simulink model "mass_springg"  (R2021a)
settings: Solver=VariableStepAuto  StartTime=0.0  StopTime=25  MaxStep=0.005  RelTol=1e-3
values from neighbouring files (symbols this model uses):
  A = adj    [ceren_function.m]    (also in deneme.m = [A_1 ;A_2; A_3;A_4; A_5;A_6])
  B = [B_1; B_2; B_3; B_4; B_5; B_6]    [deneme.m]
  B_dist = 2*[0; 0.0717; 0; -0.7374; 0; 1.9776]    [deneme.m]
  C1 = [0.0717 0 -0.7374 0 1.9776 0]    [deneme.m]
  C2 = [0.0699 0 -0.5958 0 1.2029 0]    [deneme.m]
  C3 = [0.0665 0 -0.4444 0 0.4020 0]    [deneme.m]
  C4 = [0.0630 0 -0.2977 0 -0.3216 0]    [deneme.m]
  D = [0 0 0 0]    [deneme.m]
  K = kron(A, B)    [kronecker.m]
  w1 = 2*pi* 0.2745    (= 1.72473436682)    [deneme.m]
  w2 = 2*pi* 2.9446    (= 18.5014674555)    [deneme.m]
settings Model: PacingRate=9  Creator=umut  LastModifiedBy=umut

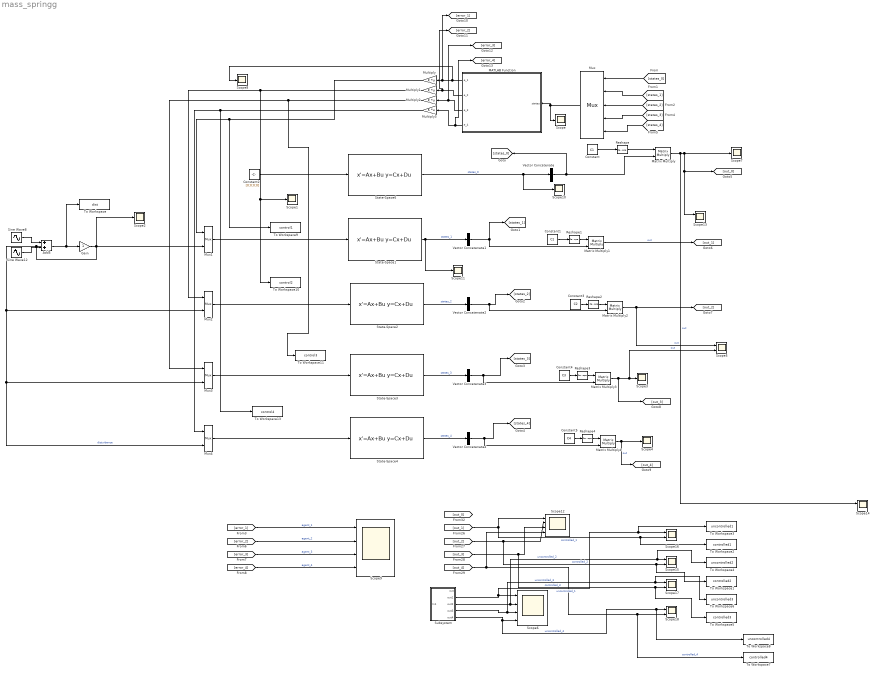
== system mass_springg ==
  Add5 : Sum
  Constant : Constant  Value=C1
  Constant1 : Constant  Value=C1
  Constant2 : Constant  Value=[0;0;0;0]
  Constant3 : Constant  Value=C2
  Constant4 : Constant  Value=C3
  Constant5 : Constant  Value=C4
  Gain : Gain
  MATLAB Function : MATLAB Function  TreatAsAtomicUnit=on
  Matrix Multiply{,1..4} (5 alike) : Product  Multiplication=Matrix(*)
  Multiply{,1..3} (4 alike) : Gain  Gain=K  Multiplication=Matrix(K*u)
  Mux : Mux  Inputs=5
  Mux{1..4} (4 alike) : Mux  Inputs=2
  Reshape{,1..4} (5 alike) : Reshape  OutputDimensionality=Customize  OutputDimensions=[1,6]
  Scope{,1..4,7..8,10..11} (9 alike) : Scope
  Scope12 : Scope  NumInputPorts=4
  Scope{5,13..18} (7 alike) : Scope  NumInputPorts=2
  Scope6 : Scope  NumInputPorts=4
  Scope9 : Scope  NumInputPorts=4
  Sine Wave12 : Sin  Amplitude=0.5  Frequency=w2  SampleTime=0
  Sine Wave8 : Sin  Amplitude=0.5  Frequency=w1  SampleTime=0
  State-Space1 : StateSpace  A=A  B=[B B_dist]  C=eye(6)  D=[D 0;D 0;D 0;D 0;D 0;D 0]  InitialCondition=[0.1;0.2;0.3;0.4;0.5;0.6]
  State-Space2 : StateSpace  A=A  B=[B B_dist]  C=eye(6)  D=[D 0;D 0;D 0;D 0;D 0;D 0]  InitialCondition=[0.6;0.5;0.4;0.3;0.2;0.1]
  State-Space3 : StateSpace  A=A  B=[B B_dist]  C=eye(6)  D=[D 0;D 0;D 0;D 0;D 0;D 0]  InitialCondition=[0.6;0.3;0.1;0.4;0;0.8]
  State-Space4 : StateSpace  A=A  B=[B B_dist]  C=eye(6)  D=[D 0;D 0;D 0;D 0;D 0;D 0]  InitialCondition=[0.3;0.1;0.7;0.2;0.8;0.4]
  State-Space6 : StateSpace  A=A  B=B  C=zeros(6)  D=[D;D;D;D;D;D]  InitialCondition=[0.1;0.2;0.3;0.4;0.5;0.6]
  Subsystem : Subsystem
  To Workspace : ToWorkspace  VariableName=dist  SampleTime=-1
      settings: Save2DSignal=2-D array (concatenate along first dimension)
  To Workspace1 : ToWorkspace  VariableName=controlled2  SampleTime=-1
      settings: Save2DSignal=2-D array (concatenate along first dimension)
  To Workspace10 : ToWorkspace  VariableName=control2  SampleTime=-1
      settings: Save2DSignal=2-D array (concatenate along first dimension)
  To Workspace11 : ToWorkspace  VariableName=control3  SampleTime=-1
      settings: Save2DSignal=2-D array (concatenate along first dimension)
  To Workspace13 : ToWorkspace  VariableName=control4  SampleTime=-1
      settings: Save2DSignal=2-D array (concatenate along first dimension)
  To Workspace2 : ToWorkspace  VariableName=controlled1  SampleTime=-1
      settings: Save2DSignal=2-D array (concatenate along first dimension)
  To Workspace3 : ToWorkspace  VariableName=uncontrolled1  SampleTime=-1
      settings: Save2DSignal=2-D array (concatenate along first dimension)
  To Workspace4 : ToWorkspace  VariableName=uncontrolled2  SampleTime=-1
      settings: Save2DSignal=2-D array (concatenate along first dimension)
  To Workspace5 : ToWorkspace  VariableName=controlled3  SampleTime=-1
      settings: Save2DSignal=2-D array (concatenate along first dimension)
  To Workspace6 : ToWorkspace  VariableName=uncontrolled3  SampleTime=-1
      settings: Save2DSignal=2-D array (concatenate along first dimension)
  To Workspace7 : ToWorkspace  VariableName=controlled4  SampleTime=-1
      settings: Save2DSignal=2-D array (concatenate along first dimension)
  To Workspace8 : ToWorkspace  VariableName=uncontrolled4  SampleTime=-1
      settings: Save2DSignal=2-D array (concatenate along first dimension)
  To Workspace9 : ToWorkspace  VariableName=control1  SampleTime=-1
      settings: Save2DSignal=2-D array (concatenate along first dimension)
  Vector Concatenate{,1..4} (5 alike) : Concatenate  NumInputs=1  Mode=Multidimensional array  ConcatenateDimension=4
  wires:
  State-Space1/1 -> Vector Concatenate1/1, Scope11/1  "states_1"
  Mux/1 -> Scope/1, MATLAB Function/1(states)
  State-Space2/1 -> Vector Concatenate2/1  "states_2"
  Matrix Multiply2/1 -> [out_2], Scope5/1  "out"
  Matrix Multiply3/1 -> [out_3], Scope5/2, Scope3/1  "out"
  State-Space3/1 -> Vector Concatenate3/1  "states_3"
  Matrix Multiply4/1 -> [out_4], Scope4/1  "out"
  State-Space4/1 -> Vector Concatenate4/1  "states_4"
  [states_0] -> Mux/1
  [states_1] -> Mux/2
  [states_4] -> Mux/5
  [states_3] -> Mux/4
  [states_2] -> Mux/3
  MATLAB Function/1(e_1) -> Scope8/1, [error_1], Multiply/1
  MATLAB Function/2(e_2) -> [error_2], Multiply1/1
  MATLAB Function/3(e_3) -> [error_3], Multiply2/1
  MATLAB Function/4(e_4) -> [error_4], Multiply3/1
  Constant/1 -> Reshape/1
  State-Space6/1 -> Scope10/1, Vector Concatenate/1  "states_0"
  Constant2/1 -> State-Space6/1
  Vector Concatenate/1 -> [states_0], Matrix Multiply/2
  Matrix Multiply/1 -> Scope14/1, [out_0], Scope13/1, Scope7/1  "out"
  Vector Concatenate1/1 -> Matrix Multiply1/2, [states_1]
  Vector Concatenate2/1 -> Matrix Multiply2/2, [states_2]
  Vector Concatenate3/1 -> Matrix Multiply3/2, [states_3]
  Vector Concatenate4/1 -> Matrix Multiply4/2, [states_4]
  Constant1/1 -> Reshape1/1
  Constant3/1 -> Reshape2/1
  Constant4/1 -> Reshape3/1
  Constant5/1 -> Reshape4/1
  Reshape/1 -> Matrix Multiply/1
  Reshape1/1 -> Matrix Multiply1/1
  Reshape2/1 -> Matrix Multiply2/1
  Reshape3/1 -> Matrix Multiply3/1
  Reshape4/1 -> Matrix Multiply4/1
  [out_1] -> Scope12/1, To Workspace2/1, Scope16/2  "controlled_1"
  [out_2] -> To Workspace1/1, Scope15/2, Scope12/2  "controlled_2"
  Subsystem/2(out1) -> To Workspace3/1, Scope16/1, Scope6/1  "uncontrolled_1"
  Subsystem/3(out2) -> To Workspace4/1, Scope15/1, Scope6/2  "uncontrolled_2"
  Subsystem/4(out3) -> To Workspace6/1, Scope17/1, Scope6/3  "uncontrolled_3"
  Subsystem/5(out4) -> To Workspace8/1, Scope18/1, Scope6/4  "uncontrolled_4"
  [out_3] -> To Workspace5/1, Scope17/2, Scope12/3  "controlled_3"
  [out_4] -> To Workspace7/1, Scope18/2, Scope12/4  "controlled_4"
  Matrix Multiply1/1 -> [out_1]  "out"
  Mux1/1 -> State-Space1/1
  Mux2/1 -> State-Space2/1
  Mux3/1 -> State-Space3/1
  Mux4/1 -> State-Space4/1
  Multiply/1 -> To Workspace9/1, Mux1/1
  Multiply1/1 -> Scope1/1, To Workspace10/1, Mux2/1
  Multiply2/1 -> To Workspace11/1, Mux3/1
  Multiply3/1 -> Mux4/1, To Workspace13/1
  Sine Wave12/1 -> Add5/2
  Sine Wave8/1 -> Add5/1
  Add5/1 -> To Workspace/1, Gain/1
  Gain/1 -> Scope2/1, Mux4/2, Mux3/2, Mux2/2, Mux1/2  "disturbance"
  [error_3] -> Scope9/3  "agent_3"
  [error_2] -> Scope9/2  "agent_2"
  [error_4] -> Scope9/4  "agent_4"
  [error_1] -> Scope9/1  "agent_1"

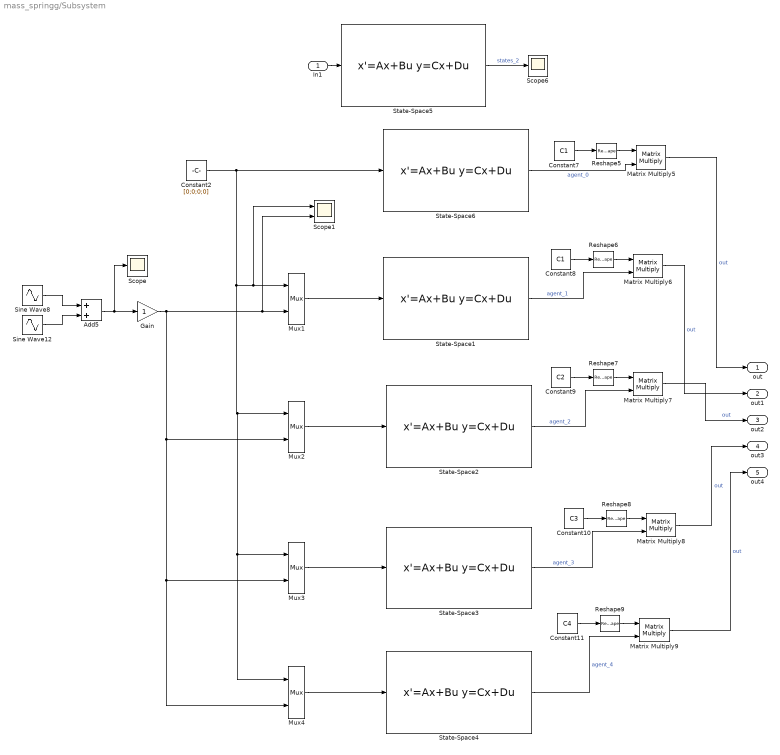
== system mass_springg/Subsystem ==
  In1 : Inport
  Add5 : Sum
  Constant10 : Constant  Value=C3
  Constant11 : Constant  Value=C4
  Constant2 : Constant  Value=[0;0;0;0]
  Constant7 : Constant  Value=C1
  Constant8 : Constant  Value=C1
  Constant9 : Constant  Value=C2
  Gain : Gain
  Matrix Multiply{5..9} (5 alike) : Product  Multiplication=Matrix(*)
  Mux{1..4} (4 alike) : Mux  Inputs=2
  Reshape{5..9} (5 alike) : Reshape  OutputDimensionality=Customize  OutputDimensions=[1,6]
  Scope : Scope
  Scope1 : Scope  NumInputPorts=2
  Scope6 : Scope
  Sine Wave12 : Sin  Amplitude=0.5  Frequency=w2  SampleTime=0
  Sine Wave8 : Sin  Amplitude=0.5  Frequency=w1  SampleTime=0
  State-Space1 : StateSpace  A=A  B=[B B_dist]  C=eye(6)  D=[D 0;D 0;D 0;D 0;D 0;D 0]  InitialCondition=[0.1;0.2;0.3;0.4;0.5;0.6]
  State-Space2 : StateSpace  A=A  B=[B B_dist]  C=eye(6)  D=[D 0;D 0;D 0;D 0;D 0;D 0]  InitialCondition=[0.6;0.5;0.4;0.3;0.2;0.1]
  State-Space3 : StateSpace  A=A  B=[B B_dist]  C=eye(6)  D=[D 0;D 0;D 0;D 0;D 0;D 0]  InitialCondition=[0.6;0.3;0.1;0.4;0;0.8]
  State-Space4 : StateSpace  A=A  B=[B B_dist]  C=eye(6)  D=[D 0;D 0;D 0;D 0;D 0;D 0]  InitialCondition=[0.3;0.1;0.7;0.2;0.8;0.4]
  State-Space5 : StateSpace  A=A  B=B  C=eye(6)  D=[D;D;D;D;D;D]  InitialCondition=[1,2,3,4,5,6]
  State-Space6 : StateSpace  A=A  B=B  C=eye(6)  D=[D;D;D;D;D;D]  InitialCondition=[0.1;0.2;0.3;0.4;0.5;0.6]
  out : Outport
  out1 : Outport  Port=2
  out2 : Outport  Port=3
  out3 : Outport  Port=4
  out4 : Outport  Port=5
  wires:
  State-Space2/1 -> Matrix Multiply7/2  "agent_2"
  Constant11/1 -> Reshape9/1
  Constant7/1 -> Reshape5/1
  State-Space3/1 -> Matrix Multiply8/2  "agent_3"
  Matrix Multiply8/1 -> out3/1  "out"
  Matrix Multiply9/1 -> out4/1  "out"
  Reshape8/1 -> Matrix Multiply8/1
  Constant9/1 -> Reshape7/1
  In1/1 -> State-Space5/1
  Reshape5/1 -> Matrix Multiply5/1
  State-Space4/1 -> Matrix Multiply9/2  "agent_4"
  State-Space1/1 -> Matrix Multiply6/2  "agent_1"
  Matrix Multiply7/1 -> out2/1  "out"
  Reshape6/1 -> Matrix Multiply6/1
  Constant8/1 -> Reshape6/1
  State-Space5/1 -> Scope6/1  "states_2"
  Matrix Multiply6/1 -> out1/1  "out"
  Constant10/1 -> Reshape8/1
  Reshape9/1 -> Matrix Multiply9/1
  Matrix Multiply5/1 -> out/1  "out"
  Reshape7/1 -> Matrix Multiply7/1
  State-Space6/1 -> Matrix Multiply5/2  "agent_0"
  Mux4/1 -> State-Space4/1
  Mux3/1 -> State-Space3/1
  Sine Wave12/1 -> Add5/2
  Sine Wave8/1 -> Add5/1
  Mux1/1 -> State-Space1/1
  Mux2/1 -> State-Space2/1
  Add5/1 -> Gain/1, Scope/1
  Constant2/1 -> Mux4/1, Mux3/1, Mux2/1, Scope1/1, Mux1/1, State-Space6/1
  Gain/1 -> Mux4/2, Mux3/2, Mux2/2, Scope1/2, Mux1/2

== matlab function mass_springg/MATLAB Function ==
  data: states input; e_1 output size=[6, 1]; e_2 output size=[6, 1]; e_3 output size=[6, 1]; e_4 output size=[6, 1]
function [e_1, e_2, e_3, e_4]  = calculate_neighborhood_error(states)
    adj = [ 0	1	1	1
            1   0   1   1
            1   1   0   1
            1   1   1   0]
    
    pinnings = [1; 0; 0; 0];

    A = adj;
    G = pinnings;
    
    size_agents = 4;
    size_states = 6;
    
    error = zeros(size_states, size_agents);
    
    
    for i = 1 : size_agents
        error_temp = [0;0;0;0;0;0];
        for j = 1 : size_agents
            error_temp = error_temp + A(i, j) * (states((j)*6+1 : 6*(j+1)) - states((i)*6+1 : 6*(i+1)));
        end
        error_temp = error_temp + pinnings(i) * (states(1 : 6) - states((i)*6+1 : 6*(i+1)));
        error(:,i) = error_temp;
    end
    
    e_1 = error(:,1);
    e_2 = error(:,2);
    e_3 = error(:,3);
    e_4 = error(:,4);
end
